simulink model "sampleModel65"  (Simulink 9.1)
settings: Solver=VariableStepAuto  StartTime=0.0  StopTime=10.0  RelTol=1e-3
undefined symbols (not defined in the file): Newton, Raphson
libraries: simulink x17
settings Model: Creator=DELL  LastModifiedBy=DELL
settings DataIOCC: SaveFormat=Dataset
settings OptimizationCC: LifeSpan=auto
settings DebuggingCC: UnderspecifiedInitializationDetection=Simplified  MergeDetectMultiDrivingBlocksExec=error  SFUnexpectedBacktrackingDiag=error  SFNoUnconditionalDefaultTransitionDiag=error  SFExecutionAtInitializationDiag=warning
settings HardwareCC: ProdBitPerPointer=64  ProdBitPerSizeT=64  ProdBitPerPtrDiffT=64  ProdLargestAtomicFloat=Float  ProdIntDivRoundTo=Zero  ProdEndianess=LittleEndian  ProdWordSize=64  ProdHWDeviceType=Intel->x86-64 (Windows64)
settings ModelReferenceCC: PropagateSignalLabelsOutOfModel=on
settings CodeAppCC: StateflowObjectComments=off
settings GRTTargetCC: TargetLangStandard=C99 (ISO)  CombineOutputUpdateFcns=on  GRTInterface=off
settings ConfigComp: CovMetricSettings=dwe  CovHtmlReporting=off  CovSaveCumulativeToWorkspaceVar=off  CovSaveSingleToWorkspaceVar=off  CovExternalEMLEnable=on

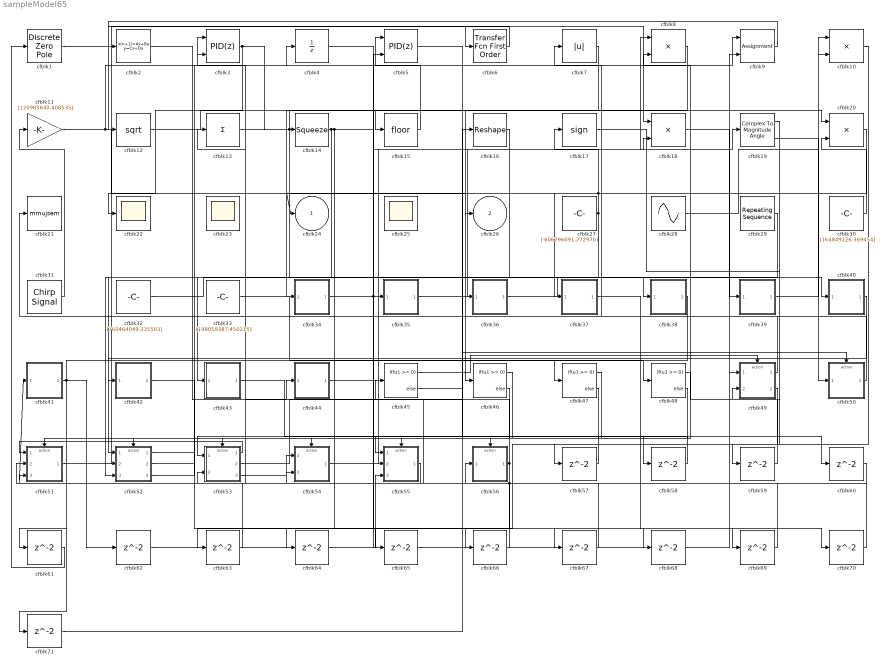
== system sampleModel65 ==
  cfblk1 : DiscreteZeroPole  Poles=[0 0.5]  Gain=1
  cfblk10 : Product  Inputs=**
  cfblk11 : Gain  Gain=[120985640.408535]
  cfblk12 : Sqrt  SaturateOnIntegerOverflow=on
  cfblk13 : Sum  Inputs=+
  cfblk14 : Squeeze
  cfblk15 : Rounding
  cfblk16 : Reshape
  cfblk17 : Signum
  cfblk18 : Product  Inputs=**
  cfblk19 : ComplexToMagnitudeAngle
  cfblk2 : DiscreteStateSpace
  cfblk20 : Product  Inputs=**
  cfblk21 : ToWorkspace  VariableName=mmujsem  SaveFormat=Timeseries  SampleTime=-1
  cfblk22 : Scope
  cfblk23 : Scope
      settings: Floating=on
  cfblk25 : Scope
      settings: Floating=on
  cfblk27 : Constant  Value=[-606796091.272970]  SampleTime=1
  cfblk28 : Sin  Amplitude=[354373032.820353]  Bias=[794142706.525440]  SampleTime=0
  cfblk29 : simulink/Sources/Repeating Sequence  rep_seq_t=[0 2]  rep_seq_y=[204516926.923834, -480250250.999293]
  cfblk3 : simulink/Continuous/PID Controller (2DOF)  Controller=PID  TimeDomain=Discrete-time  SampleTime=1  IntegratorMethod=Forward Euler  FilterMethod=Forward Euler  Form=Parallel  UseFilter=on  ControllerParametersSource=internal  P=1  I=1  D=0  N=100  b=1  c=1  InitialConditionSource=internal  InitialConditionForIntegrator=0  InitialConditionForFilter=0  ExternalReset=none  LimitOutput=off  UpperSaturationLimit=inf  LowerSaturationLimit=-inf  LinearizeAsGain=off  AntiWindupMode=none  Kb=1  TrackingMode=off  Kt=1  PParamMin=[]  PParamMax=[]  IParamMin=[]  IParamMax=[]  DParamMin=[]  DParamMax=[]  NParamMin=[]  NParamMax=[]  bParamMin=[]  bParamMax=[]  cParamMin=[]  cParamMax=[]  KbParamMin=[]  KbParamMax=[]  KtParamMin=[]  KtParamMax=[]  POutMin=[]  POutMax=[]  IOutMin=[]  IOutMax=[]  DOutMin=[]  DOutMax=[]  NOutMin=[]  NOutMax=[]  bOutMin=[]  bOutMax=[]  cOutMin=[]  cOutMax=[]  KbOutMin=[]  KbOutMax=[]  KtOutMin=[]  KtOutMax=[]  IntegratorOutMin=[]  IntegratorOutMax=[]  FilterOutMin=[]  FilterOutMax=[]  SumOutMin=[]  SumOutMax=[]  Sum1OutMin=[]  Sum1OutMax=[]  Sum2OutMin=[]  Sum2OutMax=[]  Sum3OutMin=[]  Sum3OutMax=[]  SumI1OutMin=[]  SumI1OutMax=[]  SumI2OutMin=[]  SumI2OutMax=[]  SumI3OutMin=[]  SumI3OutMax=[]  SumDOutMin=[]  SumDOutMax=[]  SaturationOutMin=[]  SaturationOutMax=[]  IntegratorContinuousStateAttributes=''  IntegratorStateMustResolveToSignalObject=off  IntegratorRTWStateStorageClass=Auto  FilterContinuousStateAttributes=''  FilterStateMustResolveToSignalObject=off  FilterRTWStateStorageClass=Auto  DifferentiatorICPrevScaledInput=0  DifferentiatorOutMin=[]  DifferentiatorOutMax=[]  FilterDiffOutCoefMin=[]  FilterDiffOutCoefMax=[]  SumDenOutMin=[]  SumDenOutMax=[]  SumNumOutMin=[]  SumNumOutMax=[]  ReciprocalOutMin=[]  ReciprocalOutMax=[]  DivideOutMin=[]  DivideOutMax=[]  TunerSelectOption=Transfer Function Based (PID Tuner App)
  cfblk30 : Constant  Value=[164849226.369454]  SampleTime=1
  cfblk31 : simulink/Sources/Chirp Signal  f1=[736637363.119903]  T=[351565025.666785]  f2=[214864807.277247]
  cfblk32 : Constant  Value=[760464049.335503]  SampleTime=1
  cfblk33 : Constant  Value=[198059387.450215]  SampleTime=1
  cfblk34 : Subsystem
  cfblk35 : Subsystem
  cfblk36 : Subsystem
  cfblk37 : Subsystem
  cfblk38 : Subsystem
  cfblk39 : Subsystem
  cfblk4 : UnitDelay
  cfblk40 : Subsystem
  cfblk41 : Subsystem
  cfblk42 : Subsystem
  cfblk43 : Subsystem
  cfblk44 : Subsystem
  cfblk{45..48} (4 alike) : If  IfExpression=u1 >= 0  SampleTime=1
  cfblk49 : Subsystem  TreatAsAtomicUnit=on
  cfblk5 : simulink/Continuous/PID Controller (2DOF)  Controller=PID  TimeDomain=Discrete-time  SampleTime=1  IntegratorMethod=Forward Euler  FilterMethod=Forward Euler  Form=Parallel  UseFilter=on  ControllerParametersSource=internal  P=1  I=1  D=0  N=100  b=1  c=1  InitialConditionSource=internal  InitialConditionForIntegrator=0  InitialConditionForFilter=0  ExternalReset=none  LimitOutput=off  UpperSaturationLimit=inf  LowerSaturationLimit=-inf  LinearizeAsGain=off  AntiWindupMode=none  Kb=1  TrackingMode=off  Kt=1  PParamMin=[]  PParamMax=[]  IParamMin=[]  IParamMax=[]  DParamMin=[]  DParamMax=[]  NParamMin=[]  NParamMax=[]  bParamMin=[]  bParamMax=[]  cParamMin=[]  cParamMax=[]  KbParamMin=[]  KbParamMax=[]  KtParamMin=[]  KtParamMax=[]  POutMin=[]  POutMax=[]  IOutMin=[]  IOutMax=[]  DOutMin=[]  DOutMax=[]  NOutMin=[]  NOutMax=[]  bOutMin=[]  bOutMax=[]  cOutMin=[]  cOutMax=[]  KbOutMin=[]  KbOutMax=[]  KtOutMin=[]  KtOutMax=[]  IntegratorOutMin=[]  IntegratorOutMax=[]  FilterOutMin=[]  FilterOutMax=[]  SumOutMin=[]  SumOutMax=[]  Sum1OutMin=[]  Sum1OutMax=[]  Sum2OutMin=[]  Sum2OutMax=[]  Sum3OutMin=[]  Sum3OutMax=[]  SumI1OutMin=[]  SumI1OutMax=[]  SumI2OutMin=[]  SumI2OutMax=[]  SumI3OutMin=[]  SumI3OutMax=[]  SumDOutMin=[]  SumDOutMax=[]  SaturationOutMin=[]  SaturationOutMax=[]  IntegratorContinuousStateAttributes=''  IntegratorStateMustResolveToSignalObject=off  IntegratorRTWStateStorageClass=Auto  FilterContinuousStateAttributes=''  FilterStateMustResolveToSignalObject=off  FilterRTWStateStorageClass=Auto  DifferentiatorICPrevScaledInput=0  DifferentiatorOutMin=[]  DifferentiatorOutMax=[]  FilterDiffOutCoefMin=[]  FilterDiffOutCoefMax=[]  SumDenOutMin=[]  SumDenOutMax=[]  SumNumOutMin=[]  SumNumOutMax=[]  ReciprocalOutMin=[]  ReciprocalOutMax=[]  DivideOutMin=[]  DivideOutMax=[]  TunerSelectOption=Transfer Function Based (PID Tuner App)
  cfblk50 : Subsystem  TreatAsAtomicUnit=on
  cfblk51 : Subsystem  TreatAsAtomicUnit=on
  cfblk52 : Subsystem  TreatAsAtomicUnit=on
  cfblk53 : Subsystem  TreatAsAtomicUnit=on
  cfblk54 : Subsystem  TreatAsAtomicUnit=on
  cfblk55 : Subsystem  TreatAsAtomicUnit=on
  cfblk56 : Subsystem  TreatAsAtomicUnit=on
  cfblk{57..71} (15 alike) : Delay  SampleTime=1
  cfblk6 : simulink/Discrete/Transfer Fcn First Order  PoleZ=0.95  ICPrevOutput=0.0  DoSatur=off
      settings: SourceProductName=Simulink
  cfblk7 : Abs
  cfblk8 : Product
  cfblk9 : Assignment  DiagnosticForDimensions=Warning  IndexOptions=Index vector (dialog)  Indices=1  OutputSizes=1
  cfblk24 : Outport
  cfblk26 : Outport  Port=2
  wires:
  cfblk41/1(cfblk2) -> cfblk61/1, cfblk62/1
  cfblk36/1(cfblk2) -> cfblk38/1(cfblk1)
  cfblk16/1 -> cfblk43/1(cfblk1)
  cfblk7/1 -> cfblk46/1
  cfblk2/1 -> cfblk44/1(cfblk1)
  cfblk51/1(cfblk2) -> cfblk18/1
  cfblk17/1 -> cfblk49/2(cfblk14)
  cfblk20/1 -> cfblk37/1(cfblk1)
  cfblk35/1(cfblk2) -> cfblk19/1
  cfblk12/1 -> cfblk15/1
  cfblk27/1 -> cfblk17/1, cfblk24/1, cfblk52/3(cfblk15)
  cfblk33/1 -> cfblk47/1
  cfblk32/1 -> cfblk40/1(cfblk1)
  cfblk11/1 -> cfblk26/1, cfblk3/1
  cfblk18/1 -> cfblk39/1(cfblk1)
  cfblk56/1(cfblk2) -> cfblk41/1(cfblk1), cfblk63/1, cfblk3/2
  cfblk50/1(cfblk2) -> cfblk7/1
  cfblk13/1 -> cfblk20/1, cfblk55/2(cfblk15)
  cfblk54/1(cfblk2) -> cfblk8/1
  cfblk44/1(cfblk2) -> cfblk48/1
  cfblk15/1 -> cfblk5/1
  cfblk9/1 -> cfblk12/1
  cfblk28/1 -> cfblk10/1
  cfblk3/1 -> cfblk22/1, cfblk14/1
  cfblk30/1 -> cfblk20/2
  cfblk49/1(cfblk2) -> cfblk21/1
  cfblk8/1 -> cfblk34/1(cfblk1)
  cfblk1/1 -> cfblk6/1
  cfblk14/1 -> cfblk18/2, cfblk64/1, cfblk42/1(cfblk1)
  cfblk34/1(cfblk2) -> cfblk35/1(cfblk1), cfblk69/1
  cfblk31/1 -> cfblk11/1
  cfblk39/1(cfblk2) -> cfblk10/2
  cfblk53/1(cfblk2) -> cfblk51/1(cfblk1)
  cfblk40/1(cfblk2) -> cfblk52/1(cfblk1)
  cfblk6/1 -> cfblk2/1
  cfblk55/1(cfblk2) -> cfblk53/2(cfblk14)
  cfblk52/1(cfblk2) -> cfblk9/1
  cfblk29/1 -> cfblk52/2(cfblk14)
  cfblk52/3(cfblk17) -> cfblk4/1
  cfblk53/2(cfblk15) -> cfblk16/1
  cfblk19/2 -> cfblk50/1(cfblk1)
  cfblk53/3(cfblk16) -> cfblk54/1(cfblk1)
  cfblk45/1 -> cfblk49/Action
  cfblk45/2 -> cfblk50/Action
  cfblk46/1 -> cfblk51/Action
  cfblk46/2 -> cfblk52/Action
  cfblk47/1 -> cfblk53/Action
  cfblk47/2 -> cfblk54/Action
  cfblk48/1 -> cfblk55/Action
  cfblk48/2 -> cfblk56/Action
  cfblk10/1 -> cfblk57/1
  cfblk57/1 -> cfblk55/1(cfblk1)
  cfblk43/1(cfblk2) -> cfblk58/1
  cfblk58/1 -> cfblk53/1(cfblk1)
  cfblk19/1 -> cfblk59/1
  cfblk59/1 -> cfblk8/2
  cfblk5/1 -> cfblk60/1
  cfblk60/1 -> cfblk56/1(cfblk1)
  cfblk61/1 -> cfblk1/1
  cfblk62/1 -> cfblk55/3(cfblk16)
  cfblk63/1 -> cfblk51/3(cfblk10)
  cfblk64/1 -> cfblk5/2
  cfblk42/1(cfblk2) -> cfblk65/1
  cfblk65/1 -> cfblk9/2
  cfblk49/2(cfblk15) -> cfblk66/1
  cfblk66/1 -> cfblk51/2(cfblk9)
  cfblk52/2(cfblk16) -> cfblk67/1
  cfblk67/1 -> cfblk45/1
  cfblk4/1 -> cfblk68/1
  cfblk68/1 -> cfblk49/1(cfblk1)
  cfblk69/1 -> cfblk54/2(cfblk11)
  cfblk37/1(cfblk2) -> cfblk70/1
  cfblk70/1 -> cfblk13/1
  cfblk38/1(cfblk2) -> cfblk71/1
  cfblk71/1 -> cfblk36/1(cfblk1)

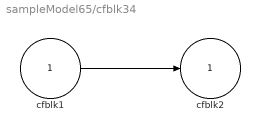
== system sampleModel65/cfblk34 ==
  cfblk1 : Inport
  cfblk2 : Outport
  wires:
  cfblk1/1 -> cfblk2/1

== system sampleModel65/cfblk35 ==
  cfblk1 : Inport
  cfblk2 : Outport
  wires:
  cfblk1/1 -> cfblk2/1

== system sampleModel65/cfblk36 ==
  cfblk1 : Inport
  cfblk2 : Outport
  wires:
  cfblk1/1 -> cfblk2/1

== system sampleModel65/cfblk37 ==
  cfblk1 : Inport
  cfblk2 : Outport
  wires:
  cfblk1/1 -> cfblk2/1

== system sampleModel65/cfblk38 ==
  cfblk1 : Inport
  cfblk2 : Outport
  wires:
  cfblk1/1 -> cfblk2/1

== system sampleModel65/cfblk39 ==
  cfblk1 : Inport
  cfblk2 : Outport
  wires:
  cfblk1/1 -> cfblk2/1

== system sampleModel65/cfblk40 ==
  cfblk1 : Inport
  cfblk2 : Outport
  wires:
  cfblk1/1 -> cfblk2/1

== system sampleModel65/cfblk41 ==
  cfblk1 : Inport
  cfblk2 : Outport
  wires:
  cfblk1/1 -> cfblk2/1

== system sampleModel65/cfblk42 ==
  cfblk1 : Inport
  cfblk2 : Outport
  wires:
  cfblk1/1 -> cfblk2/1

== system sampleModel65/cfblk43 ==
  cfblk1 : Inport
  cfblk2 : Outport
  wires:
  cfblk1/1 -> cfblk2/1

== system sampleModel65/cfblk44 ==
  cfblk1 : Inport
  cfblk2 : Outport
  wires:
  cfblk1/1 -> cfblk2/1

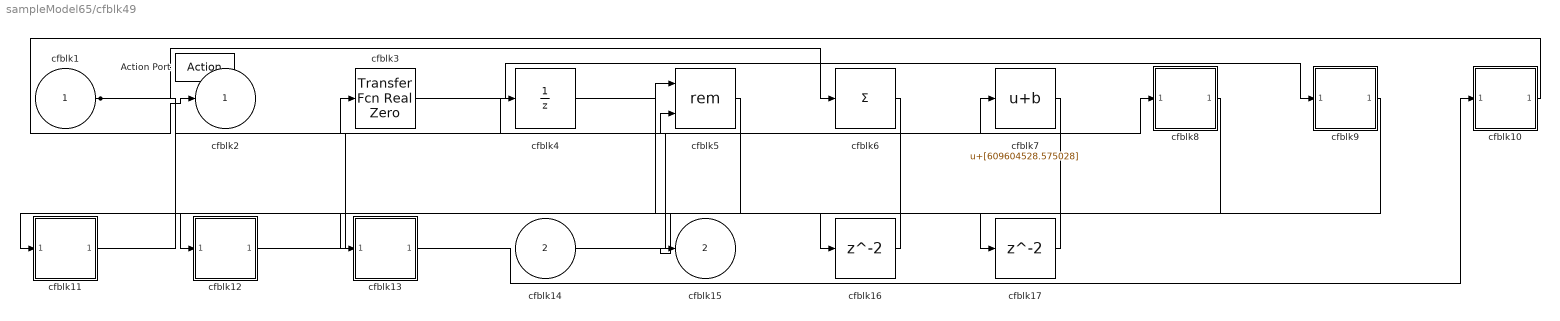
== system sampleModel65/cfblk49 ==
  cfblk1 : Inport
  cfblk14 : Inport  Port=2
  Action Port : ActionPort  ActionType=then
  cfblk10 : Subsystem
  cfblk11 : Subsystem
  cfblk12 : Subsystem
  cfblk13 : Subsystem
  cfblk16 : Delay
  cfblk17 : Delay
  cfblk3 : simulink/Discrete/Transfer Fcn Real Zero  ZeroZ=0.75  ICPrevInput=0.0  DoSatur=off
      settings: SourceProductName=Simulink  SourceProductBaseCode=SL
  cfblk4 : UnitDelay  SampleTime=-1
  cfblk5 : Math  Operator=rem  SaturateOnIntegerOverflow=on
  cfblk6 : Sum  Inputs=+
  cfblk7 : Bias  Bias=[609604528.575028]
  cfblk8 : Subsystem
  cfblk9 : Subsystem
  cfblk2 : Outport
  cfblk15 : Outport  Port=2
  wires:
  cfblk12/1(cfblk2) -> cfblk8/1(cfblk1)
  cfblk14/1 -> cfblk7/1
  cfblk1/1 -> cfblk6/1, cfblk5/2
  cfblk8/1(cfblk2) -> cfblk15/1
  cfblk7/1 -> cfblk12/1(cfblk1)
  cfblk3/1 -> cfblk9/1(cfblk1)
  cfblk11/1(cfblk2) -> cfblk4/1
  cfblk6/1 -> cfblk13/1(cfblk1)
  cfblk13/1(cfblk2) -> cfblk10/1(cfblk1)
  cfblk10/1(cfblk2) -> cfblk2/1
  cfblk5/1 -> cfblk11/1(cfblk1)
  cfblk4/1 -> cfblk16/1
  cfblk16/1 -> cfblk5/1
  cfblk9/1(cfblk2) -> cfblk17/1
  cfblk17/1 -> cfblk3/1

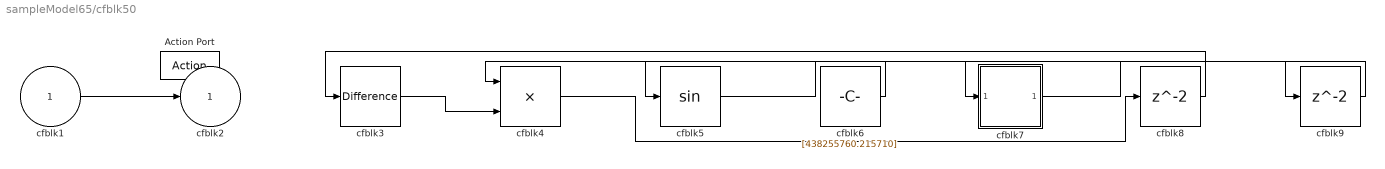
== system sampleModel65/cfblk50 ==
  cfblk1 : Inport
  Action Port : ActionPort  ActionType=else
  cfblk3 : simulink/Discrete/Difference  ICPrevInput=0.0  OutMin=[]  OutMax=[]  OutDataTypeStr=Inherit: Inherit via back propagation  OutDataType=fixdt(1, 16)  OutScaling=2^-10  DoSatur=off
  cfblk4 : Product
  cfblk5 : Trigonometry
  cfblk6 : Constant  Value=[438255760.215710]  SampleTime=1
  cfblk7 : Subsystem
  cfblk8 : Delay
  cfblk9 : Delay
  cfblk2 : Outport
  wires:
  cfblk1/1 -> cfblk2/1
  cfblk6/1 -> cfblk4/1
  cfblk3/1 -> cfblk4/2
  cfblk5/1 -> cfblk7/1(cfblk1)
  cfblk4/1 -> cfblk8/1
  cfblk8/1 -> cfblk3/1
  cfblk7/1(cfblk2) -> cfblk9/1
  cfblk9/1 -> cfblk5/1

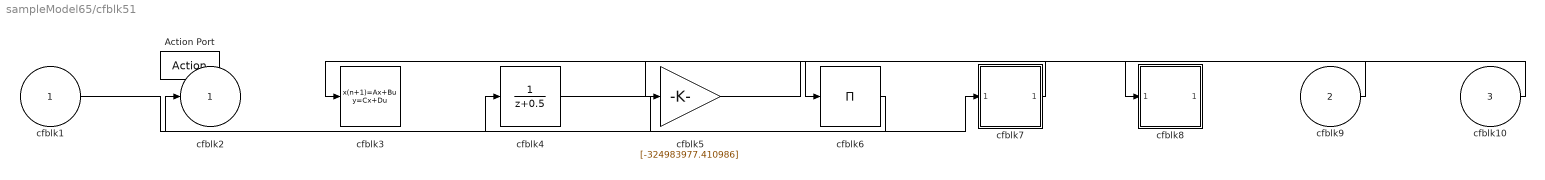
== system sampleModel65/cfblk51 ==
  cfblk1 : Inport
  cfblk9 : Inport  Port=2
  cfblk10 : Inport  Port=3
  Action Port : ActionPort  ActionType=then
  cfblk3 : DiscreteStateSpace  SampleTime=-1
  cfblk4 : DiscreteTransferFcn
  cfblk5 : Gain  Gain=[-324983977.410986]
  cfblk6 : Product  Inputs=*
  cfblk7 : Subsystem
  cfblk8 : Subsystem
  cfblk2 : Outport
  wires:
  cfblk10/1 -> cfblk6/1
  cfblk4/1 -> cfblk7/1(cfblk1)
  cfblk5/1 -> cfblk8/1(cfblk1)
  cfblk6/1 -> cfblk2/1
  cfblk7/1(cfblk2) -> cfblk3/1
  cfblk1/1 -> cfblk4/1
  cfblk9/1 -> cfblk5/1

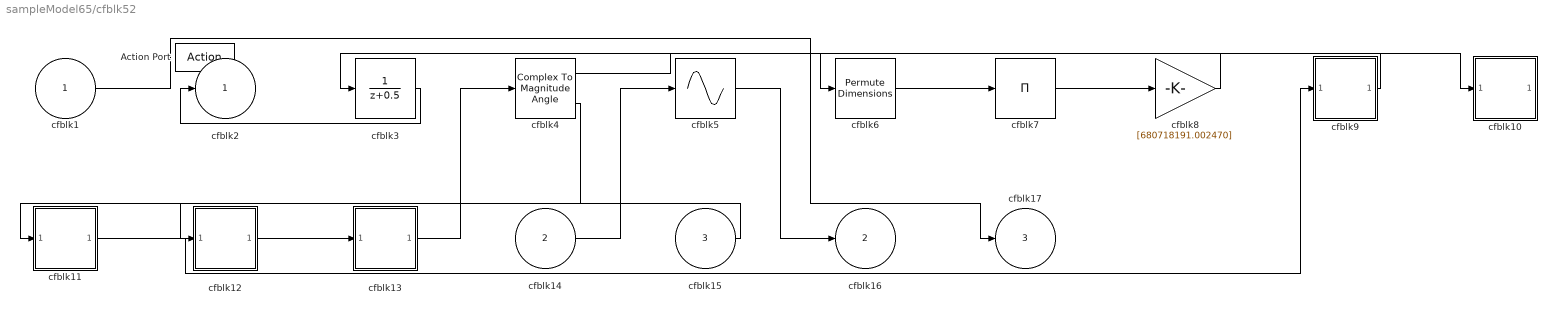
== system sampleModel65/cfblk52 ==
  cfblk1 : Inport
  cfblk14 : Inport  Port=2
  cfblk15 : Inport  Port=3
  Action Port : ActionPort  ActionType=else
  cfblk10 : Subsystem
  cfblk11 : Subsystem
  cfblk12 : Subsystem
  cfblk13 : Subsystem
  cfblk3 : DiscreteTransferFcn
  cfblk4 : ComplexToMagnitudeAngle
  cfblk5 : Sin  TimeSource=Use external signal  SampleTime=0
  cfblk6 : PermuteDimensions
  cfblk7 : Product  Inputs=*
  cfblk8 : Gain  Gain=[680718191.002470]
  cfblk9 : Subsystem
  cfblk2 : Outport
  cfblk16 : Outport  Port=2
  cfblk17 : Outport  Port=3
  wires:
  cfblk9/1(cfblk2) -> cfblk6/1
  cfblk12/1(cfblk2) -> cfblk13/1(cfblk1)
  cfblk3/1 -> cfblk2/1
  cfblk14/1 -> cfblk5/1
  cfblk6/1 -> cfblk7/1
  cfblk7/1 -> cfblk8/1
  cfblk13/1(cfblk2) -> cfblk4/1
  cfblk11/1(cfblk2) -> cfblk9/1(cfblk1)
  cfblk1/1 -> cfblk17/1
  cfblk5/1 -> cfblk16/1
  cfblk8/1 -> cfblk3/1
  cfblk4/1 -> cfblk10/1(cfblk1)
  cfblk15/1 -> cfblk12/1(cfblk1)
  cfblk4/2 -> cfblk11/1(cfblk1)

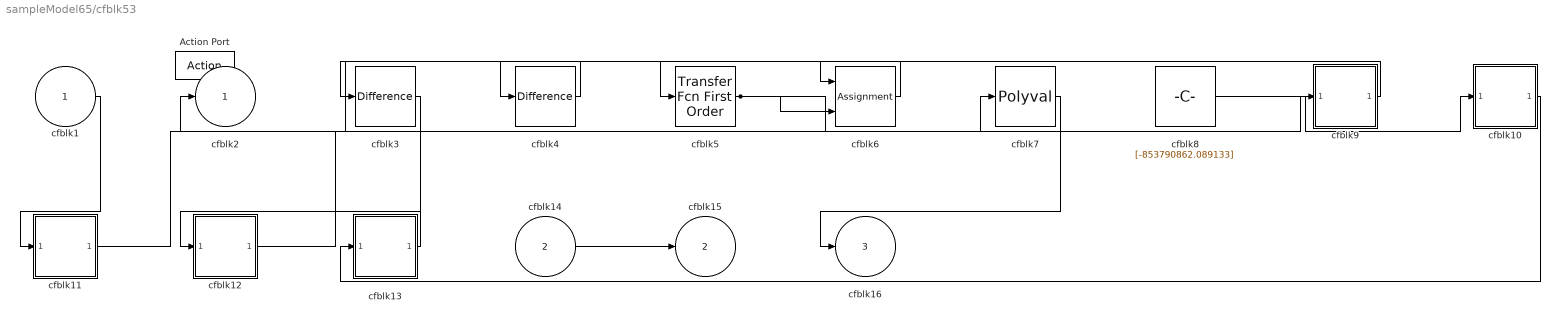
== system sampleModel65/cfblk53 ==
  cfblk1 : Inport
  cfblk14 : Inport  Port=2
  Action Port : ActionPort  ActionType=then
  cfblk10 : Subsystem
  cfblk11 : Subsystem
  cfblk12 : Subsystem
  cfblk13 : Subsystem
  cfblk3 : simulink/Discrete/Difference  ICPrevInput=0.0  OutMin=[]  OutMax=[]  OutDataTypeStr=Inherit: Inherit via back propagation  OutDataType=fixdt(1, 16)  OutScaling=2^-10  DoSatur=off
  cfblk4 : simulink/Discrete/Difference  ICPrevInput=0.0  OutMin=[]  OutMax=[]  OutDataTypeStr=Inherit: Inherit via back propagation  OutDataType=fixdt(1, 16)  OutScaling=2^-10  DoSatur=off
  cfblk5 : simulink/Discrete/Transfer Fcn First Order  PoleZ=0.95  ICPrevOutput=0.0  DoSatur=off
      settings: SourceProductName=Simulink
  cfblk6 : Assignment  DiagnosticForDimensions=Warning  IndexOptions=Index vector (dialog)  Indices=1  OutputSizes=1
  cfblk7 : Polyval  Coefs=[ +2.081618890e-019, -1.441693666e-014, +4.719686976e-010, -8.536869453e-006, +1.621573104e-001, -8.087801117e+001 ]
  cfblk8 : Constant  Value=[-853790862.089133]  SampleTime=1
  cfblk9 : Subsystem
  cfblk2 : Outport
  cfblk15 : Outport  Port=2
  cfblk16 : Outport  Port=3
  wires:
  cfblk3/1 -> cfblk12/1(cfblk1)
  cfblk9/1(cfblk2) -> cfblk6/1
  cfblk11/1(cfblk2) -> cfblk5/1
  cfblk14/1 -> cfblk15/1
  cfblk10/1(cfblk2) -> cfblk13/1(cfblk1)
  cfblk8/1 -> cfblk10/1(cfblk1)
  cfblk12/1(cfblk2) -> cfblk7/1
  cfblk6/1 -> cfblk4/1
  cfblk7/1 -> cfblk16/1
  cfblk5/1 -> cfblk9/1(cfblk1), cfblk6/2
  cfblk1/1 -> cfblk11/1(cfblk1)
  cfblk4/1 -> cfblk3/1
  cfblk13/1(cfblk2) -> cfblk2/1

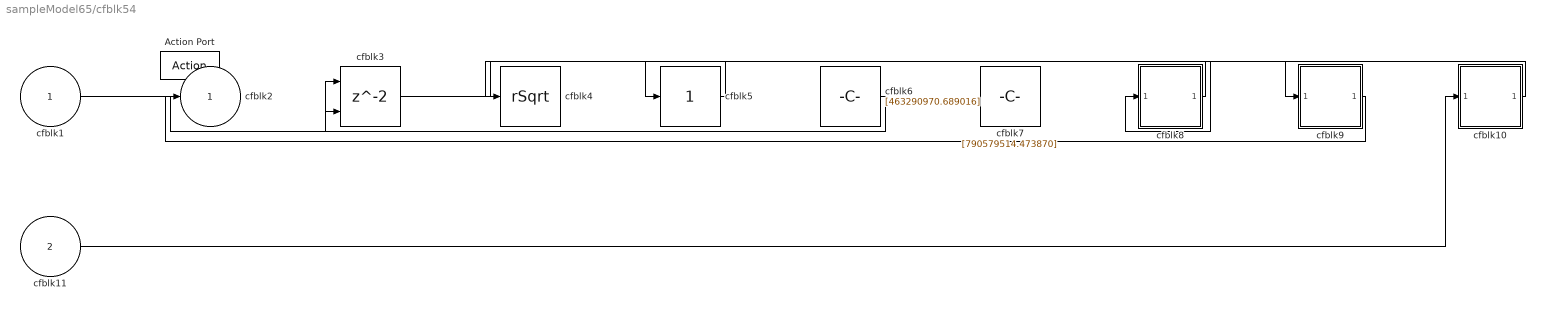
== system sampleModel65/cfblk54 ==
  cfblk1 : Inport
  cfblk11 : Inport  Port=2
  Action Port : ActionPort  ActionType=else
  cfblk10 : Subsystem
  cfblk3 : Delay  ShowEnablePort=on
      settings: InputPortMap=u0,e6
  cfblk4 : Sqrt  Operator=rSqrt  AlgorithmType=Newton-Raphson  SaturateOnIntegerOverflow=on
  cfblk5 : simulink/Math Operations/Slider Gain  gain=1  low=0  high=2
  cfblk6 : Constant  Value=[463290970.689016]  SampleTime=1
  cfblk7 : Constant  Value=[790579514.473870]  SampleTime=1
  cfblk8 : Subsystem
  cfblk9 : Subsystem
  cfblk2 : Outport
  wires:
  cfblk1/1 -> cfblk3/1
  cfblk6/1 -> cfblk3/2
  cfblk11/1 -> cfblk10/1(cfblk1)
  cfblk8/1(cfblk2) -> cfblk5/1
  cfblk10/1(cfblk2) -> cfblk8/1(cfblk1)
  cfblk3/1 -> cfblk9/1(cfblk1)
  cfblk5/1 -> cfblk4/1
  cfblk9/1(cfblk2) -> cfblk2/1

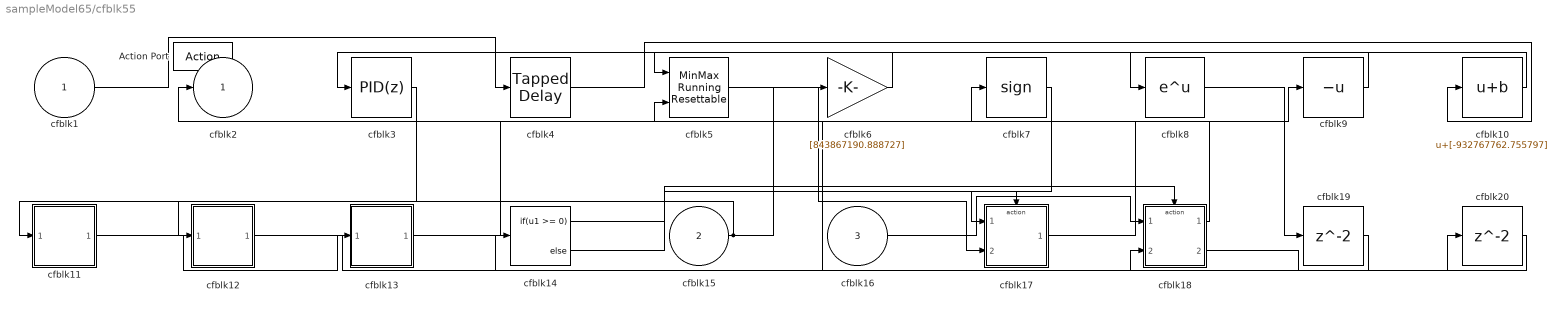
== system sampleModel65/cfblk55 ==
  cfblk1 : Inport
  cfblk15 : Inport  Port=2
  cfblk16 : Inport  Port=3
  Action Port : ActionPort  ActionType=then
  cfblk10 : Bias  Bias=[-932767762.755797]
  cfblk11 : Subsystem
  cfblk12 : Subsystem
  cfblk13 : Subsystem
  cfblk14 : If  IfExpression=u1 >= 0  SampleTime=1
  cfblk17 : Subsystem  TreatAsAtomicUnit=on
  cfblk18 : Subsystem  TreatAsAtomicUnit=on
  cfblk19 : Delay
  cfblk20 : Delay
  cfblk3 : simulink/Continuous/PID Controller  Controller=PID  TimeDomain=Discrete-time  SampleTime=-1  IntegratorMethod=Forward Euler  FilterMethod=Forward Euler  Form=Parallel  UseFilter=on  ControllerParametersSource=internal  P=1  I=1  D=0  N=100  InitialConditionSource=internal  InitialConditionForIntegrator=0  InitialConditionForFilter=0  ExternalReset=none  LimitOutput=off  UpperSaturationLimit=inf  LowerSaturationLimit=-inf  LinearizeAsGain=off  AntiWindupMode=none  Kb=1  TrackingMode=off  Kt=1  PParamMin=[]  PParamMax=[]  IParamMin=[]  IParamMax=[]  DParamMin=[]  DParamMax=[]  NParamMin=[]  NParamMax=[]  KbParamMin=[]  KbParamMax=[]  KtParamMin=[]  KtParamMax=[]  POutMin=[]  POutMax=[]  IOutMin=[]  IOutMax=[]  DOutMin=[]  DOutMax=[]  NOutMin=[]  NOutMax=[]  KbOutMin=[]  KbOutMax=[]  KtOutMin=[]  KtOutMax=[]  IntegratorOutMin=[]  IntegratorOutMax=[]  FilterOutMin=[]  FilterOutMax=[]  SumOutMin=[]  SumOutMax=[]  SumI1OutMin=[]  SumI1OutMax=[]  SumI2OutMin=[]  SumI2OutMax=[]  SumI3OutMin=[]  SumI3OutMax=[]  SumDOutMin=[]  SumDOutMax=[]  SaturationOutMin=[]  SaturationOutMax=[]  IntegratorContinuousStateAttributes=''  IntegratorStateMustResolveToSignalObject=off  IntegratorRTWStateStorageClass=Auto  FilterContinuousStateAttributes=''  FilterStateMustResolveToSignalObject=off  FilterRTWStateStorageClass=Auto  DifferentiatorICPrevScaledInput=0  DifferentiatorOutMin=[]  DifferentiatorOutMax=[]  FilterDiffOutCoefMin=[]  FilterDiffOutCoefMax=[]  SumDenOutMin=[]  SumDenOutMax=[]  SumNumOutMin=[]  SumNumOutMax=[]  ReciprocalOutMin=[]  ReciprocalOutMax=[]  DivideOutMin=[]  DivideOutMax=[]  TunerSelectOption=Transfer Function Based (PID Tuner App)
  cfblk4 : simulink/Discrete/Tapped Delay  vinit=0.0  samptime=-1  NumDelays=1  DelayOrder=Oldest  includeCurrent=off
  cfblk5 : simulink/Math Operations/MinMax Running Resettable  Function=min  vinit=0.0
  cfblk6 : Gain  Gain=[843867190.888727]
  cfblk7 : Signum
  cfblk8 : Math  SaturateOnIntegerOverflow=on
  cfblk9 : UnaryMinus
  cfblk2 : Outport
  wires:
  cfblk10/1 -> cfblk5/1
  cfblk17/1(cfblk2) -> cfblk9/1
  cfblk16/1 -> cfblk18/1(cfblk1)
  cfblk9/1 -> cfblk8/1
  cfblk3/1 -> cfblk11/1(cfblk1)
  cfblk13/1(cfblk2) -> cfblk5/2
  cfblk4/1 -> cfblk10/1
  cfblk12/1(cfblk2) -> cfblk7/1
  cfblk11/1(cfblk2) -> cfblk13/1(cfblk1)
  cfblk1/1 -> cfblk4/1
  cfblk7/1 -> cfblk17/1(cfblk1)
  cfblk6/1 -> cfblk3/1
  cfblk18/1(cfblk2) -> cfblk2/1
  cfblk5/1 -> cfblk17/2(cfblk14)
  cfblk15/1 -> cfblk12/1(cfblk1), cfblk6/1
  cfblk14/1 -> cfblk17/Action
  cfblk14/2 -> cfblk18/Action
  cfblk8/1 -> cfblk19/1
  cfblk19/1 -> cfblk18/2(cfblk10)
  cfblk18/2(cfblk11) -> cfblk20/1
  cfblk20/1 -> cfblk14/1

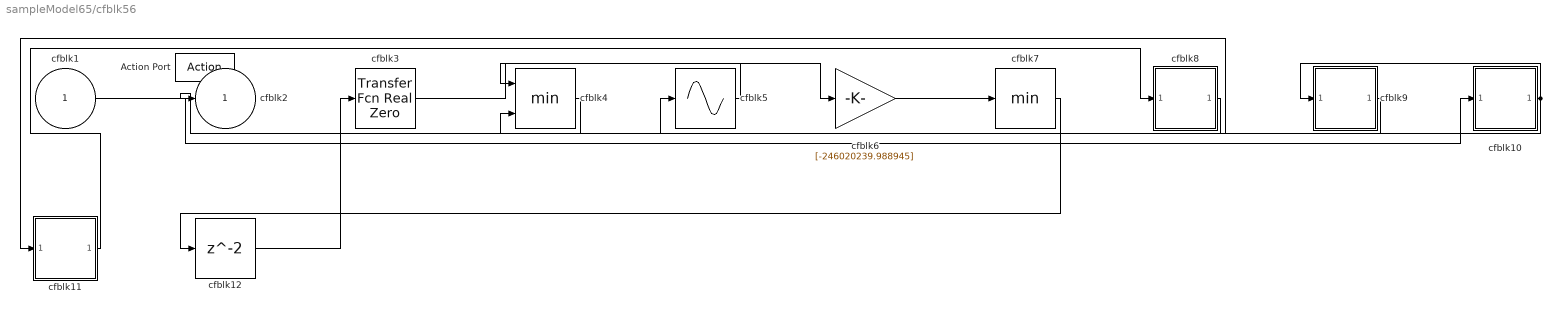
== system sampleModel65/cfblk56 ==
  cfblk1 : Inport
  Action Port : ActionPort  ActionType=else
  cfblk10 : Subsystem
  cfblk11 : Subsystem
  cfblk12 : Delay
  cfblk3 : simulink/Discrete/Transfer Fcn Real Zero  ZeroZ=0.75  ICPrevInput=0.0  DoSatur=off
      settings: SourceProductName=Simulink  SourceProductBaseCode=SL
  cfblk4 : MinMax  Inputs=2
  cfblk5 : Sin  TimeSource=Use external signal  SampleTime=0
  cfblk6 : Gain  Gain=[-246020239.988945]
  cfblk7 : MinMax
  cfblk8 : Subsystem
  cfblk9 : Subsystem
  cfblk2 : Outport
  wires:
  cfblk10/1(cfblk2) -> cfblk9/1(cfblk1), cfblk4/2
  cfblk3/1 -> cfblk6/1
  cfblk8/1(cfblk2) -> cfblk5/1
  cfblk1/1 -> cfblk10/1(cfblk1)
  cfblk11/1(cfblk2) -> cfblk8/1(cfblk1)
  cfblk9/1(cfblk2) -> cfblk11/1(cfblk1)
  cfblk5/1 -> cfblk4/1
  cfblk6/1 -> cfblk7/1
  cfblk4/1 -> cfblk2/1
  cfblk7/1 -> cfblk12/1
  cfblk12/1 -> cfblk3/1

== system sampleModel65/cfblk49/cfblk10 ==
  cfblk1 : Inport
  cfblk2 : Outport
  wires:
  cfblk1/1 -> cfblk2/1

== system sampleModel65/cfblk49/cfblk11 ==
  cfblk1 : Inport
  cfblk2 : Outport
  wires:
  cfblk1/1 -> cfblk2/1

== system sampleModel65/cfblk49/cfblk12 ==
  cfblk1 : Inport
  cfblk2 : Outport
  wires:
  cfblk1/1 -> cfblk2/1

== system sampleModel65/cfblk49/cfblk13 ==
  cfblk1 : Inport
  cfblk2 : Outport
  wires:
  cfblk1/1 -> cfblk2/1

== system sampleModel65/cfblk49/cfblk8 ==
  cfblk1 : Inport
  cfblk2 : Outport
  wires:
  cfblk1/1 -> cfblk2/1

== system sampleModel65/cfblk49/cfblk9 ==
  cfblk1 : Inport
  cfblk2 : Outport
  wires:
  cfblk1/1 -> cfblk2/1

== system sampleModel65/cfblk50/cfblk7 ==
  cfblk1 : Inport
  cfblk2 : Outport
  wires:
  cfblk1/1 -> cfblk2/1

== system sampleModel65/cfblk51/cfblk7 ==
  cfblk1 : Inport
  cfblk2 : Outport
  wires:
  cfblk1/1 -> cfblk2/1

== system sampleModel65/cfblk51/cfblk8 ==
  cfblk1 : Inport
  cfblk2 : Outport
  wires:
  cfblk1/1 -> cfblk2/1

== system sampleModel65/cfblk52/cfblk10 ==
  cfblk1 : Inport
  cfblk2 : Outport
  wires:
  cfblk1/1 -> cfblk2/1

== system sampleModel65/cfblk52/cfblk11 ==
  cfblk1 : Inport
  cfblk2 : Outport
  wires:
  cfblk1/1 -> cfblk2/1

== system sampleModel65/cfblk52/cfblk12 ==
  cfblk1 : Inport
  cfblk2 : Outport
  wires:
  cfblk1/1 -> cfblk2/1

== system sampleModel65/cfblk52/cfblk13 ==
  cfblk1 : Inport
  cfblk2 : Outport
  wires:
  cfblk1/1 -> cfblk2/1

== system sampleModel65/cfblk52/cfblk9 ==
  cfblk1 : Inport
  cfblk2 : Outport
  wires:
  cfblk1/1 -> cfblk2/1

== system sampleModel65/cfblk53/cfblk10 ==
  cfblk1 : Inport
  cfblk2 : Outport
  wires:
  cfblk1/1 -> cfblk2/1

== system sampleModel65/cfblk53/cfblk11 ==
  cfblk1 : Inport
  cfblk2 : Outport
  wires:
  cfblk1/1 -> cfblk2/1

== system sampleModel65/cfblk53/cfblk12 ==
  cfblk1 : Inport
  cfblk2 : Outport
  wires:
  cfblk1/1 -> cfblk2/1

== system sampleModel65/cfblk53/cfblk13 ==
  cfblk1 : Inport
  cfblk2 : Outport
  wires:
  cfblk1/1 -> cfblk2/1

== system sampleModel65/cfblk53/cfblk9 ==
  cfblk1 : Inport
  cfblk2 : Outport
  wires:
  cfblk1/1 -> cfblk2/1

== system sampleModel65/cfblk54/cfblk10 ==
  cfblk1 : Inport
  cfblk2 : Outport
  wires:
  cfblk1/1 -> cfblk2/1

== system sampleModel65/cfblk54/cfblk8 ==
  cfblk1 : Inport
  cfblk2 : Outport
  wires:
  cfblk1/1 -> cfblk2/1

== system sampleModel65/cfblk54/cfblk9 ==
  cfblk1 : Inport
  cfblk2 : Outport
  wires:
  cfblk1/1 -> cfblk2/1

== system sampleModel65/cfblk55/cfblk11 ==
  cfblk1 : Inport
  cfblk2 : Outport
  wires:
  cfblk1/1 -> cfblk2/1

== system sampleModel65/cfblk55/cfblk12 ==
  cfblk1 : Inport
  cfblk2 : Outport
  wires:
  cfblk1/1 -> cfblk2/1

== system sampleModel65/cfblk55/cfblk13 ==
  cfblk1 : Inport
  cfblk2 : Outport
  wires:
  cfblk1/1 -> cfblk2/1

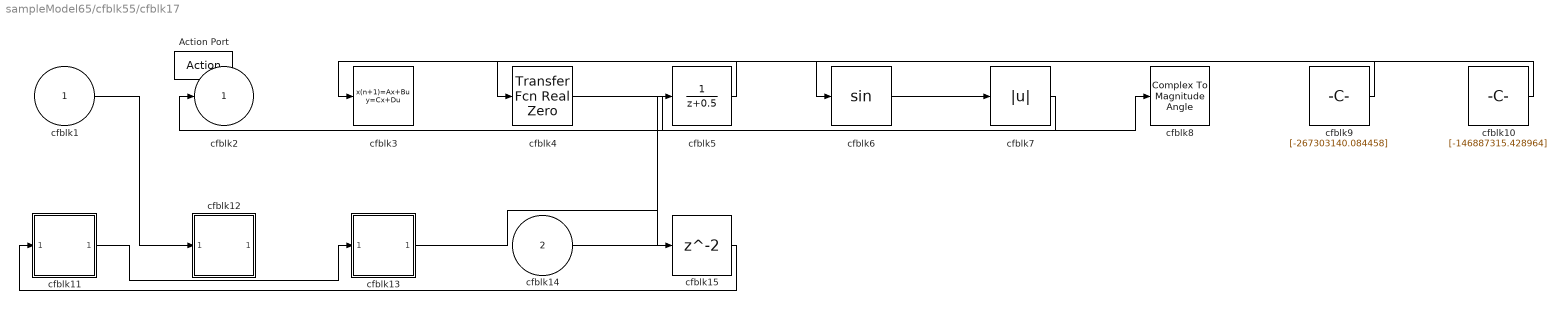
== system sampleModel65/cfblk55/cfblk17 ==
  cfblk1 : Inport
  cfblk14 : Inport  Port=2
  Action Port : ActionPort  ActionType=then
  cfblk10 : Constant  Value=[-146887315.428964]  SampleTime=1
  cfblk11 : Subsystem
  cfblk12 : Subsystem
  cfblk13 : Subsystem
  cfblk15 : Delay
  cfblk3 : DiscreteStateSpace  SampleTime=-1
  cfblk4 : simulink/Discrete/Transfer Fcn Real Zero  ZeroZ=0.75  ICPrevInput=0.0  DoSatur=off
      settings: SourceProductName=Simulink  SourceProductBaseCode=SL
  cfblk5 : DiscreteTransferFcn
  cfblk6 : Trigonometry
  cfblk7 : Abs
  cfblk8 : ComplexToMagnitudeAngle
  cfblk9 : Constant  Value=[-267303140.084458]  SampleTime=1
  cfblk2 : Outport
  wires:
  cfblk1/1 -> cfblk12/1(cfblk1)
  cfblk9/1 -> cfblk3/1
  cfblk4/1 -> cfblk8/1
  cfblk14/1 -> cfblk5/1
  cfblk11/1(cfblk2) -> cfblk13/1(cfblk1)
  cfblk7/1 -> cfblk2/1
  cfblk5/1 -> cfblk4/1
  cfblk6/1 -> cfblk7/1
  cfblk10/1 -> cfblk6/1
  cfblk13/1(cfblk2) -> cfblk15/1
  cfblk15/1 -> cfblk11/1(cfblk1)

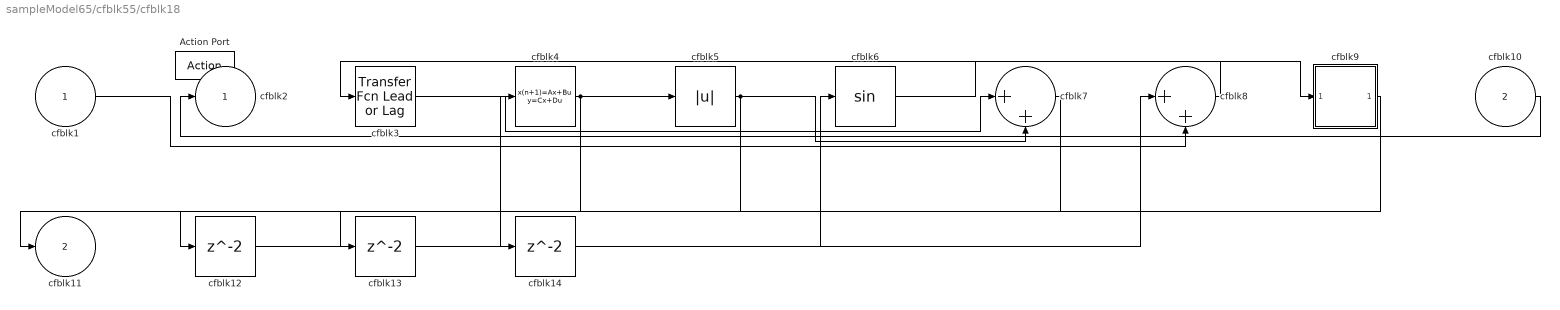
== system sampleModel65/cfblk55/cfblk18 ==
  cfblk1 : Inport
  cfblk10 : Inport  Port=2
  Action Port : ActionPort  ActionType=else
  cfblk12 : Delay
  cfblk13 : Delay
  cfblk14 : Delay
  cfblk3 : simulink/Discrete/Transfer Fcn Lead or Lag  PoleZ=0.95  ZeroZ=0.75  ICPrevOutput=0.0  ICPrevInput=0.0  DoSatur=off
      settings: SourceProductName=Simulink  SourceProductBaseCode=SL
  cfblk4 : DiscreteStateSpace  SampleTime=-1
  cfblk5 : Abs
  cfblk6 : Trigonometry
  cfblk7 : Sum  Inputs=|++
  cfblk8 : Sum  Inputs=|++
  cfblk9 : Subsystem
  cfblk2 : Outport
  cfblk11 : Outport  Port=2
  wires:
  cfblk10/1 -> cfblk2/1
  cfblk3/1 -> cfblk7/1
  cfblk6/1 -> cfblk9/1(cfblk1)
  cfblk5/1 -> cfblk7/2, cfblk13/1
  cfblk8/1 -> cfblk3/1
  cfblk4/1 -> cfblk5/1, cfblk11/1
  cfblk1/1 -> cfblk8/2
  cfblk7/1 -> cfblk12/1
  cfblk12/1 -> cfblk8/1
  cfblk13/1 -> cfblk4/1
  cfblk9/1(cfblk2) -> cfblk14/1
  cfblk14/1 -> cfblk6/1

== system sampleModel65/cfblk56/cfblk10 ==
  cfblk1 : Inport
  cfblk2 : Outport
  wires:
  cfblk1/1 -> cfblk2/1

== system sampleModel65/cfblk56/cfblk11 ==
  cfblk1 : Inport
  cfblk2 : Outport
  wires:
  cfblk1/1 -> cfblk2/1

== system sampleModel65/cfblk56/cfblk8 ==
  cfblk1 : Inport
  cfblk2 : Outport
  wires:
  cfblk1/1 -> cfblk2/1

== system sampleModel65/cfblk56/cfblk9 ==
  cfblk1 : Inport
  cfblk2 : Outport
  wires:
  cfblk1/1 -> cfblk2/1

== system sampleModel65/cfblk55/cfblk17/cfblk11 ==
  cfblk1 : Inport
  cfblk2 : Outport
  wires:
  cfblk1/1 -> cfblk2/1

== system sampleModel65/cfblk55/cfblk17/cfblk12 ==
  cfblk1 : Inport
  cfblk2 : Outport
  wires:
  cfblk1/1 -> cfblk2/1

== system sampleModel65/cfblk55/cfblk17/cfblk13 ==
  cfblk1 : Inport
  cfblk2 : Outport
  wires:
  cfblk1/1 -> cfblk2/1

== system sampleModel65/cfblk55/cfblk18/cfblk9 ==
  cfblk1 : Inport
  cfblk2 : Outport
  wires:
  cfblk1/1 -> cfblk2/1
